simulink model "untitled"  (R2023a)
settings: Solver=VariableStepAuto  StartTime=0.0  StopTime=0.1  RelTol=1e-3
libraries: spsCurrentMeasurementLib x4, spsThyristorLib x4, spsVoltageMeasurementLib x3, spsACVoltageSourceLib x1, spsSeriesRLCBranchLib x1, sps_lib x1
settings Model: Creator=付  LastModifiedBy=付

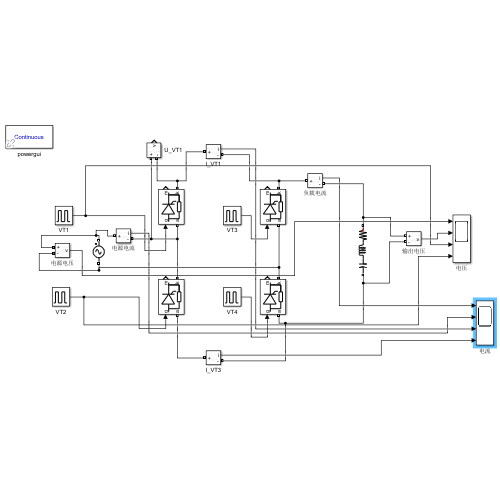
[thumbnail: Simulink's stored preview of the top-level diagram]
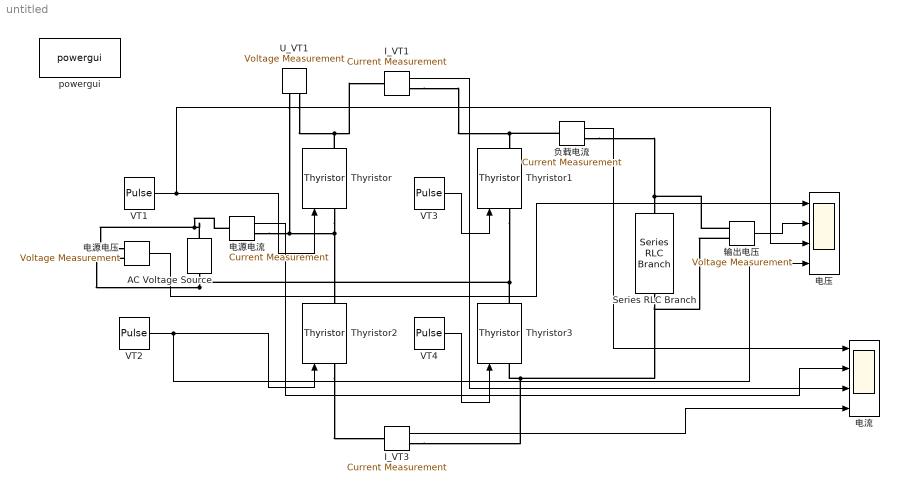
== system untitled ==
  AC Voltage Source : spsACVoltageSourceLib/AC Voltage Source  Amplitude=100  Phase=0  Frequency=50  SampleTime=0  Measurements=None  BusType=swing  Pref=10e3  Qref=0  Qmin=-inf  Qmax=+inf
  I_VT1 : spsCurrentMeasurementLib/Current Measurement  PhasorSimulation=off  OutputType=Complex  PSBequivalent=0
  I_VT3 : spsCurrentMeasurementLib/Current Measurement  PhasorSimulation=off  OutputType=Complex  PSBequivalent=0
  Series RLC Branch : spsSeriesRLCBranchLib/Series RLC Branch  LConnTagsString=__new0  RConnTagsString=__new0  BranchType=RLC  Resistance=30  Inductance=1e-5  SetiL0=off  InitialCurrent=0  Capacitance=0  Setx0=off  InitialVoltage=0  Measurements=None
  Thyristor{,1..3} (4 alike) : spsThyristorLib/Thyristor  Ron=0.001  Lon=0  Vf=0.8  IC=0  Rs=500  Cs=250e-9  Measurements=on
  U_VT1 : spsVoltageMeasurementLib/Voltage Measurement  PhasorSimulation=off  OutputType=Complex  PSBequivalent=0
  VT1 : DiscretePulseGenerator  PulseType=Time based  Period=0.02  PulseWidth=2  PhaseDelay=30*0.02/360
  VT2 : DiscretePulseGenerator  PulseType=Time based  Period=0.02  PulseWidth=2  PhaseDelay=220*0.02/360
  VT3 : DiscretePulseGenerator  PulseType=Time based  Period=0.02  PulseWidth=2  PhaseDelay=220*0.02/360
  VT4 : DiscretePulseGenerator  PulseType=Time based  Period=0.02  PulseWidth=2  PhaseDelay=30*0.02/360
  powergui : sps_lib/powergui  Priority=1  SimulationMode=Continuous  SampleTime=50e-6  frequency=60  Iterations=50  frequencyindice=50  Pbase=100e6  ErrMax=1e-4  UnitsV=kV  UnitsW=MW  buscounter=0  FunctionMessages=off  echomessages=off  EnableUseOfTLC=off  CurrentSourceSwitches=off  DisableSnubberDevices=off  DisableRonSwitches=off  DisableVfSwitches=off  DisplayEquations=off  AutomaticDiscreteSolvers=off  SolverType=Tustin/Backward Euler (TBE)  Interpol=off  ExternalGateDelay=off  methode=off  Ts=100  x0status=blocks  SPID=on  SwTol=0  HookPort=off  NonlinearTolerance=1e-4  nMaxIteration=100  ContinueOnMaxIteration=off  RestoreLinks=warning  ResistiveCurrentMeasurement=off  Frange=[0:2:500]  Ylog=off  Xlog=on  ShowGrid=off  save=off  variable=ZData  structure=0  ZoomFFT=off  StartTime=0.0  cycles=1  DisplayStyle=1  fundamental=60  FreqAxis=off  MaxFrequency=1000  frequencyindicesteady=1  RmsSteady=1  display=off
  电压 : Scope  NumInputPorts=4
  电流 : Scope  NumInputPorts=4
  电源电压 : spsVoltageMeasurementLib/Voltage Measurement  PhasorSimulation=off  OutputType=Complex  PSBequivalent=0
  电源电流 : spsCurrentMeasurementLib/Current Measurement  PhasorSimulation=off  OutputType=Complex  PSBequivalent=0
  负载电流 : spsCurrentMeasurementLib/Current Measurement  PhasorSimulation=off  OutputType=Complex  PSBequivalent=0
  输出电压 : spsVoltageMeasurementLib/Voltage Measurement  PhasorSimulation=off  OutputType=Complex  PSBequivalent=0
  wires:
  VT1/1 -> 电压/3, Thyristor/1
  VT3/1 -> Thyristor1/1
  VT4/1 -> Thyristor3/1
  VT2/1 -> 电压/4, Thyristor2/1
  电源电压/1 -> 电压/1
  输出电压/1 -> 电压/2
  负载电流/1 -> 电流/1
  电源电流/1 -> 电流/2
  I_VT1/1 -> 电流/3
  I_VT3/1 -> 电流/4
  connections:
  AC Voltage Source/RConn1 -- 电源电流/LConn1 -- 电源电压/LConn1
  输出电压/LConn2 -- Series RLC Branch/RConn1 -- I_VT3/RConn1 -- Thyristor3/LConn1
  Thyristor1/LConn1 -- Thyristor3/RConn1 -- 电源电压/LConn2 -- AC Voltage Source/LConn1
  负载电流/LConn1 -- I_VT1/RConn1 -- Thyristor1/RConn1
  负载电流/RConn1 -- 输出电压/LConn1 -- Series RLC Branch/LConn1
  电源电流/RConn1 -- U_VT1/LConn1 -- Thyristor/LConn1 -- Thyristor2/RConn1
  U_VT1/LConn2 -- Thyristor/RConn1 -- I_VT1/LConn1
  Thyristor2/LConn1 -- I_VT3/LConn1
